simulink model "Copy_3_continuos_plant"  (R2016b)
settings: Solver=ode15s  StartTime=0.0  StopTime=300  RelTol=0.01  AbsTol=0.01
undefined symbols (not defined in the file or in its folder): deg, rad, s
libraries: simulink x12, aerolibconvert2 x4, aerolib6dof2 x2, dspsrcs4 x2, dspinverses x1
(part 1 of 2)
settings Model: Creator=Utente  LastModifiedBy=liana
settings SolverCC: MaxOrder=3  MaxConsecutiveMinStep=5  SolverJacobianMethodControl=FullAnalytical  ZeroCrossControl=DisableAll
settings DataIOCC: SaveState=on
settings OptimizationCC: BlockReduction=off  DefaultParameterBehavior=Inlined  BufferReuse=off

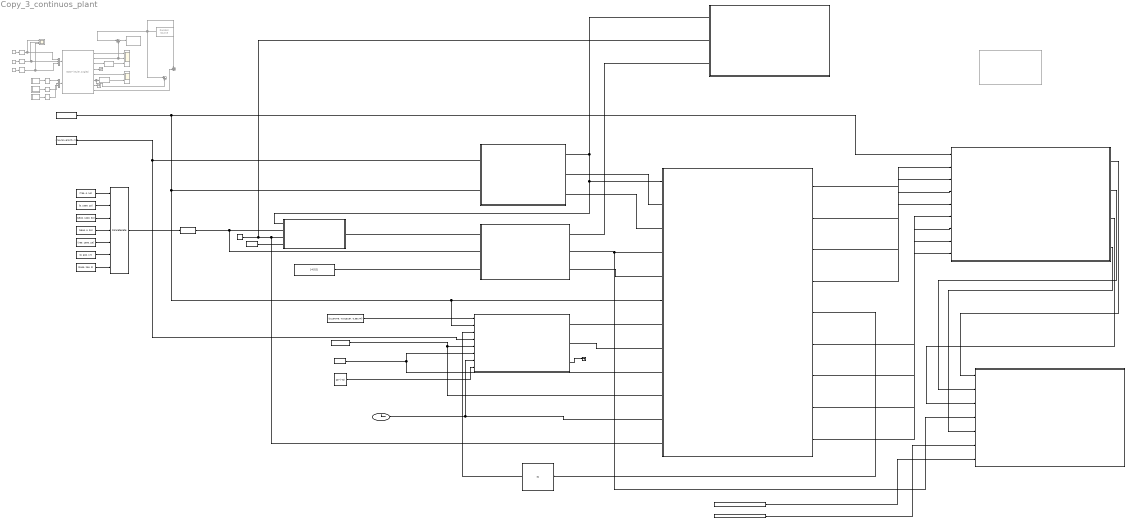
== system Copy_3_continuos_plant ==
  note: Six Degree of Freedom Motion Platform
  note: Copyright 1990-2016 The MathWorks, Inc.
  6DOF (Euler Angles) : aerolib6dof2/6DOF (Euler Angles)  Commented=on  units=Metric (MKS)  mtype=Fixed  rep=Euler Angles  xme_0=[0 0 0]  Vm_0=[0 0 0]  eul_0=[0 0 0]  pm_0=[0 0 0]  mass_0=1.0  mass_e=0.5  mass_f=2.0  inertia=eye(3)  inertia_e=eye(3)  inertia_f=2*eye(3)  k_quat=1.0  vre_flag=on
  Angle Conversion : aerolibconvert2/Angle Conversion  Commented=on  IU=rad  OU=deg
  Angular Velocity Conversion : aerolibconvert2/Angular Velocity Conversion  Commented=on  IU=rad/s  OU=deg/s
  Attitude Observer : Subsystem
  Body : Scope  Commented=on  NumInputPorts=2
  Clock : Clock
      settings: Decimation=50
  Const : Constant  Commented=on
  Const1 : Constant  Commented=on  Value=0
  Const2 : Constant  Commented=on  Value=0
  From File : FromFile  FileName=angular_velocity.mat  SampleTime=0
  From File1 : FromFile  FileName=acceleration.mat  SampleTime=0
  Fx Slider : simulink/Math Operations/Slider Gain  Commented=on  low=-1  gain=0.29496  high=1
  Fy Slider : simulink/Math Operations/Slider Gain  Commented=on  low=-1  gain=0.20144  high=1
  Fz Slider : simulink/Math Operations/Slider Gain  Commented=on  low=-1  gain=0.05036  high=1
  IC : InitialCondition  Value=[0;0;0]
  IMU data generation : Subsystem  Commented=on
  Inertial : Scope  Commented=on  NumInputPorts=3
  Kalman - Bucy Filter : Subsystem
  Kp : Constant  Value=[10 0 0; 0 10 0; 0 0 10] * 100
  Local linearization1 : Subsystem
  Math Function : Math  Operator=transpose  SaturateOnIntegerOverflow=on
  Matrix Concatenate (transponders positions) : Concatenate  NumInputs=7  Mode=Multidimensional array  ConcatenateDimension=2
  Mechanisation subsystem : Subsystem
  Mux : Mux  Commented=on  Inputs=3
  Mux1 : Mux  Commented=on  Inputs=3
  Mxx Slider : simulink/Math Operations/Slider Gain  Commented=on  low=0  gain=0  high=1
  Myy Slider : simulink/Math Operations/Slider Gain  Commented=on  low=-1  gain=0  high=1
  Mzz Slider : simulink/Math Operations/Slider Gain  Commented=on  low=-1  gain=-1  high=3
  Nonlinear algebraic transform and solution : Subsystem
  Pitch moment : Subsystem  Commented=on  mask(timed input){t=[0 3 3 4 4 5 5  7.5 7.5 8.5 8.5 9.5 9.5 10], u=[0 0  1 1 -1 -1.005 0 0 -1 -1 1 1 0 0]*3.138/2}
      mask prompts: t "time values:"; u "input values"
      mask Display: plot(t,u)
  Q matrix : Constant  Value=diag([0, 0, 0, 10^-5, 10^-3, 10^-3, 10^-3, 10^-8, 10^-8, 10^-8])
  R matrix : Constant  Value=0.25*diag([1 1 1 1 1 1])
  Random Source : dspsrcs4/Random Source  Commented=on  SrcType=Gaussian  NormMethod=Ziggurat  CltLength=12  MinVal=0  MaxVal=1  MeanVal=[0; 0; 0]  VarVal=[0.5; 0.5; 0.5]  RepMode=Not repeatable  rawSeed=1  IsInherit=off  SampMode=Continuous  SampTime=-1  SampFrame=1  DataType=Double  OutComplex=Real  OutputFrames=off
  Roll moment : Subsystem  Commented=on  mask(timed input){t=[0 1 1 2 2  10], u=[1 1 -1 -.998  0 0]*3.144/2}
      mask prompts: t "time values:"; u "input values"
      mask Display: plot(t,u)
  Scope : Scope  Commented=on  NumInputPorts=3
  Sum1 : Sum  Commented=on  Inputs=|++
  Sum2 : Sum  Commented=on  Inputs=++|
  Sum3 : Sum  Commented=on  Inputs=|++
  Terminator : Terminator
  Terminator1 : Terminator  Commented=on
  Terminator3 : Terminator  Commented=on
  Translational Motion Observer : Subsystem
  Yaw moment : Subsystem  Commented=on  mask(timed input){t=[0 6 6 7 7 8 8 10], u=[0 0  -1 -1 1 1 0 0]*3.1/2}
      mask prompts: t "time values:"; u "input values"
      mask Display: plot(t,u)
  algebraic transform - error dynamics : Subsystem
  beta : Constant  Value=100
  epsilon : Constant  Value=[1 1 1 1 1 1 1]*0.1
  ki : Constant  Value=10^(-5)
  magneto_values (Pisa) : Constant  Value=[0.237976, -0.013187, 0.39174]'
  p_n_1 : Constant  Value=[750, 0, 10]
  p_n_2 : Constant  Value=[0, 1000, 15]
  p_n_3 : Constant  Value=[1500, 1000, 30]
  p_n_4 : Constant  Value=[1500, 0, 20]
  p_n_5 : Constant  Value=[750, 1000, 25]
  p_n_6 : Constant  Value=[0, 600, 17]
  p_n_7 : Constant  Value=[2000, 200, 2]
  pos_nav file : ToFile  Commented=on  Filename=position_nav.mat  MatrixName=pos_nav  SaveFormat=Timeseries
  position_0_fixed_reference : Constant  Value=[4 5 5]
  pseudorange_measurement_model : MATLAB Function  TreatAsAtomicUnit=on
  sigma : Constant  Value=0.1
  wires:
  Clock/1 -> Translational Motion Observer/11(t), Attitude Observer/7(t)
  Nonlinear algebraic transform and solution/2(delta) -> Kalman - Bucy Filter/4(sensors measurements), Translational Motion Observer/4(delta)
  Attitude Observer/1(J) -> Translational Motion Observer/7(J)
  Attitude Observer/2(R_nb_stim) -> Translational Motion Observer/8(R_nb_stim)
  Attitude Observer/3(b_stim) -> Terminator/1
  Kp/1 -> Translational Motion Observer/10(Kp), Attitude Observer/5(Kp)
  sigma/1 -> Translational Motion Observer/9(sigma), Attitude Observer/6(sigma)
  Nonlinear algebraic transform and solution/3(C_dx) -> Translational Motion Observer/5(C_dx)
  Local linearization1/1(AL) -> Kalman - Bucy Filter/1(AL)
  Local linearization1/2(BL) -> Kalman - Bucy Filter/2(BL)
  Local linearization1/3(CL) -> Kalman - Bucy Filter/3(CL)
  pseudorange_measurement_model/1(y) -> Nonlinear algebraic transform and solution/1(y)
  Local linearization1/4(U) -> Kalman - Bucy Filter/5(U)
  epsilon/1 -> pseudorange_measurement_model/4(epsilon)
  Matrix Concatenate (transponders positions)/1 -> Math Function/1
  R matrix/1 -> Kalman - Bucy Filter/6(R)
  Q matrix/1 -> Kalman - Bucy Filter/7(Q)
  Translational Motion Observer/1(K) -> Local linearization1/2(K)
  Translational Motion Observer/2("C ") -> Local linearization1/3(C)
  Translational Motion Observer/3(" A") -> Local linearization1/4(A)
  Translational Motion Observer/4(B) -> Local linearization1/5(B)
  ki/1 -> Attitude Observer/8(Ki)
  p_n_5/1 -> Matrix Concatenate (transponders positions)/5
  p_n_4/1 -> Matrix Concatenate (transponders positions)/4
  p_n_3/1 -> Matrix Concatenate (transponders positions)/3
  p_n_2/1 -> Matrix Concatenate (transponders positions)/2
  p_n_1/1 -> Matrix Concatenate (transponders positions)/1
  Math Function/1 -> Nonlinear algebraic transform and solution/2(p), pseudorange_measurement_model/2(p_n_i)
  position_0_fixed_reference/1 -> Nonlinear algebraic transform and solution/3(p0)
  magneto_values (Pisa)/1 -> Attitude Observer/1(m_b_mag)
  p_n_6/1 -> Matrix Concatenate (transponders positions)/6
  Yaw moment/1(Out1) -> Mzz Slider/1
  Pitch moment/1(Out1) -> Myy Slider/1
  Roll moment/1(Out1) -> Mxx Slider/1
  Const2/1 -> Fz Slider/1
  Const1/1 -> Fy Slider/1
  Const/1 -> Fx Slider/1
  Mux1/1 -> 6DOF (Euler Angles)/2
  Mzz Slider/1 -> Mux1/3
  Myy Slider/1 -> Mux1/2
  Mxx Slider/1 -> Mux1/1
  Mux/1 -> 6DOF (Euler Angles)/1
  Fy Slider/1 -> Scope/2, Mux/2
  Fz Slider/1 -> Scope/3, Mux/3
  Fx Slider/1 -> Scope/1, Mux/1
  6DOF (Euler Angles)/4 -> Terminator3/1
  6DOF (Euler Angles)/7 -> Terminator1/1
  6DOF (Euler Angles)/3 -> Angle Conversion/1
  6DOF (Euler Angles)/5 -> Body/1  "Velocity in Body Axes"
  6DOF (Euler Angles)/1 -> Inertial/1  "Velocity in Inertial Axes"
  6DOF (Euler Angles)/2 -> Inertial/2, Sum1/2  "Position in Inertial Axes"
  Angle Conversion/1 -> Inertial/3  "Euler Angles"
  6DOF (Euler Angles)/6 -> Sum3/2, Angular Velocity Conversion/1
  Angular Velocity Conversion/1 -> Body/2  "Body Rotational Rates"
  6DOF (Euler Angles)/8 -> Sum2/2
  Random Source/1 -> Sum3/1, Sum2/1, Sum1/1
  Sum1/1 -> pos_nav file/1
  From File/1 -> Attitude Observer/4(w_ib), Mechanisation subsystem/1(w_ib)
  From File1/1 -> Translational Motion Observer/6(f_b_imu), Attitude Observer/2(f_b), Mechanisation subsystem/2(f_b_imu), Local linearization1/1(f_b_imu)
  p_n_7/1 -> Matrix Concatenate (transponders positions)/7
  beta/1 -> algebraic transform - error dynamics/2(beta), Translational Motion Observer/12(beta_true), pseudorange_measurement_model/3(beta)
  Mechanisation subsystem/2(v_n) -> Translational Motion Observer/2(v_n_true)
  Mechanisation subsystem/3(f_n) -> Translational Motion Observer/3(f_n_true)
  Translational Motion Observer/5(f_n_stim) -> IC/1
  Mechanisation subsystem/1(p_n) -> Translational Motion Observer/1(p_n_delta_true), pseudorange_measurement_model/1(p_n), algebraic transform - error dynamics/1(p_n_true)
  Translational Motion Observer/6(p_n_delta_err) -> Local linearization1/6(p_n_err)
  Translational Motion Observer/7(beta_err) -> Local linearization1/7(beta_err)
  Translational Motion Observer/8(v_n_err) -> Local linearization1/8(v_n_err)
  Translational Motion Observer/9(f_n_err) -> Local linearization1/9(f_n_err)
  Nonlinear algebraic transform and solution/1(x_at) -> algebraic transform - error dynamics/3(x_at)
  IC/1 -> Attitude Observer/3(f_n_stim)

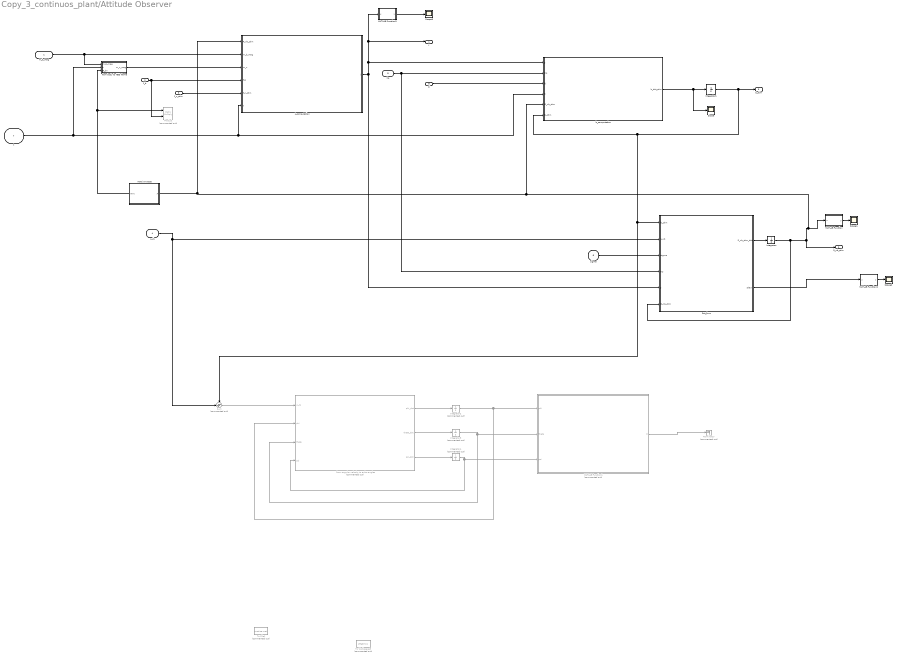
== system Copy_3_continuos_plant/Attitude Observer ==
  m_b_mag : Inport
  f_b : Inport  Port=2
  f_n_stim : Inport  Port=3
  w_ib : Inport  Port=4
  Kp : Inport  Port=5
  sigma : Inport  Port=6
  t : Inport  Port=7
  Ki : Inport  Port=8
  Integrator : Integrator  InitialCondition=eye(3)  AbsoluteTolerance=0.000000000001
  Integrator1 : Integrator  InitialCondition=0.02  UpperSaturationLimit=100  LowerSaturationLimit=-100  AbsoluteTolerance=0.0000001
  Integrator2 : Integrator  Commented=on
  Integrator3 : Integrator  Commented=on
  Integrator4 : Integrator  Commented=on
  J_computation : Subsystem
  MATLAB Function : MATLAB Function  TreatAsAtomicUnit=on
  MATLAB Function1 : MATLAB Function  Commented=on  TreatAsAtomicUnit=on
  MATLAB Function2 : MATLAB Function  TreatAsAtomicUnit=on
  MATLAB Function3 : MATLAB Function  TreatAsAtomicUnit=on
  Product : Product  Commented=on  Multiplication=Matrix(*)
  Rot_func : MATLAB Function  TreatAsAtomicUnit=on
  Scope{,1..3} (4 alike) : Scope
  Sum : Sum  Commented=on  Inputs=-+|
  Terminator : Terminator  Commented=on
  To File1 : ToFile  Commented=on  Filename=matrice.mat  MatrixName=m  SaveFormat=Timeseries
  To Workspace5 : ToWorkspace  Commented=on  VariableName=JMatrix1  SaveFormat=Timeseries  SampleTime=-1
  b_computation : MATLAB Function  TreatAsAtomicUnit=on
  from angular velocity to euler angles : MATLAB Function  Commented=on  TreatAsAtomicUnit=on
  from body to NED frame : MATLAB Function  TreatAsAtomicUnit=on
  matrixInverse : MATLAB Function  TreatAsAtomicUnit=on
  J : Outport
  R_nb_stim : Outport  Port=2
  b_stim : Outport  Port=3
  wires:
  m_b_mag/1 -> from body to NED frame/1(m_b_mag), J_computation/2(m_b_mag)
  from body to NED frame/1(m_n_mag) -> J_computation/3(m_n)
  f_b/1 -> Product/2, J_computation/4(f_b)
  J_computation/1(J) -> MATLAB Function3/1(u), J/1, b_computation/1(J), Rot_func/5(J)
  Kp/1 -> Rot_func/4(Kp), b_computation/2(Kp)
  Ki/1 -> b_computation/3(ki)
  sigma/1 -> Rot_func/3(sigma)
  w_ib/1 -> Sum/2, Rot_func/2(w_ib)
  t/1 -> from body to NED frame/2(t), b_computation/4(t), J_computation/6(t)
  b_computation/1(b_dot_stim) -> Scope/1, Integrator1/1
  matrixInverse/1(AInv) -> from body to NED frame/3(R_bn), Product/1
  MATLAB Function/1(y) -> Scope1/1
  Sum/1 -> from angular velocity to euler angles/1(w_ib)
  from angular velocity to euler angles/1(phi_dot) -> Integrator2/1
  from angular velocity to euler angles/2(theta_dot) -> Integrator3/1
  from angular velocity to euler angles/3(psi_dot) -> Integrator4/1
  Integrator3/1 -> MATLAB Function1/2(theta), from angular velocity to euler angles/3(theta)
  Integrator4/1 -> MATLAB Function1/3(psi), from angular velocity to euler angles/4(psi)
  Integrator2/1 -> from angular velocity to euler angles/2(phi), MATLAB Function1/1(phi)
  MATLAB Function2/1(y) -> Scope2/1
  Rot_func/2(Skew) -> MATLAB Function2/1(u)
  Integrator1/1 -> b_computation/6(b_stim), Sum/1, Rot_func/1(b_stim), b_stim/1
  MATLAB Function1/1(R) -> Terminator/1
  MATLAB Function3/1(y) -> Scope3/1
  Rot_func/1(R_nb_stim_dot) -> Integrator/1
  Integrator/1 -> Rot_func/6(R_nb_stim), J_computation/1(R_nb_stim), matrixInverse/1(A), b_computation/5(R_nb_stim), MATLAB Function/1(u), R_nb_stim/1
  f_n_stim/1 -> J_computation/5(f_n_stim)

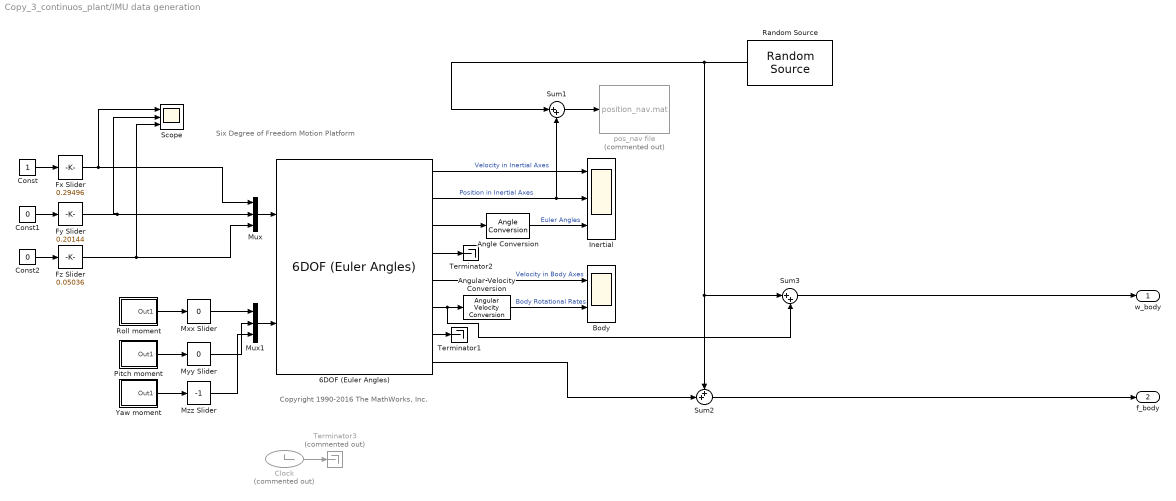
== system Copy_3_continuos_plant/IMU data generation ==
  note: Six Degree of Freedom Motion Platform
  note: Copyright 1990-2016 The MathWorks, Inc.
  6DOF (Euler Angles) : aerolib6dof2/6DOF (Euler Angles)  units=Metric (MKS)  mtype=Fixed  rep=Euler Angles  xme_0=[0 0 0]  Vm_0=[0 0 0]  eul_0=[0 0 0]  pm_0=[0 0 0]  mass_0=1.0  mass_e=0.5  mass_f=2.0  inertia=eye(3)  inertia_e=eye(3)  inertia_f=2*eye(3)  k_quat=1.0  vre_flag=on
  Angle Conversion : aerolibconvert2/Angle Conversion  IU=rad  OU=deg
  Angular Velocity Conversion : aerolibconvert2/Angular Velocity Conversion  IU=rad/s  OU=deg/s
  Body : Scope  NumInputPorts=2
  Clock : Clock  Commented=on
      settings: Decimation=100
  Const : Constant
  Const1 : Constant  Value=0
  Const2 : Constant  Value=0
  Fx Slider : simulink/Math Operations/Slider Gain  low=-1  gain=0.29496  high=1
  Fy Slider : simulink/Math Operations/Slider Gain  low=-1  gain=0.20144  high=1
  Fz Slider : simulink/Math Operations/Slider Gain  low=-1  gain=0.05036  high=1
  Inertial : Scope  NumInputPorts=3
  Mux : Mux  Inputs=3
  Mux1 : Mux  Inputs=3
  Mxx Slider : simulink/Math Operations/Slider Gain  low=0  gain=0  high=1
  Myy Slider : simulink/Math Operations/Slider Gain  low=-1  gain=0  high=1
  Mzz Slider : simulink/Math Operations/Slider Gain  low=-1  gain=-1  high=3
  Pitch moment : Subsystem  mask(timed input){t=[0 3 3 4 4 5 5  7.5 7.5 8.5 8.5 9.5 9.5 10], u=[0 0  1 1 -1 -1.005 0 0 -1 -1 1 1 0 0]*3.138/2}
      mask prompts: t "time values:"; u "input values"
      mask Display: plot(t,u)
  Random Source : dspsrcs4/Random Source  SrcType=Gaussian  NormMethod=Ziggurat  CltLength=12  MinVal=0  MaxVal=1  MeanVal=[0; 0; 0]  VarVal=[0.5; 0.5; 0.5]  RepMode=Not repeatable  rawSeed=1  IsInherit=off  SampMode=Continuous  SampTime=-1  SampFrame=1  DataType=Double  OutComplex=Real  OutputFrames=off
  Roll moment : Subsystem  mask(timed input){t=[0 1 1 2 2  10], u=[1 1 -1 -.998  0 0]*3.144/2}
      mask prompts: t "time values:"; u "input values"
      mask Display: plot(t,u)
  Scope : Scope  NumInputPorts=3
  Sum1 : Sum  Inputs=|++
  Sum2 : Sum  Inputs=++|
  Sum3 : Sum  Inputs=|++
  Terminator1 : Terminator
  Terminator2 : Terminator
  Terminator3 : Terminator  Commented=on
  Yaw moment : Subsystem  mask(timed input){t=[0 6 6 7 7 8 8 10], u=[0 0  -1 -1 1 1 0 0]*3.1/2}
      mask prompts: t "time values:"; u "input values"
      mask Display: plot(t,u)
  pos_nav file : ToFile  Commented=on  Filename=position_nav.mat  MatrixName=pos_nav  SaveFormat=Timeseries
  w_body : Outport
  f_body : Outport  Port=2
  wires:
  Yaw moment/1(Out1) -> Mzz Slider/1
  Pitch moment/1(Out1) -> Myy Slider/1
  Roll moment/1(Out1) -> Mxx Slider/1
  Const2/1 -> Fz Slider/1
  Const1/1 -> Fy Slider/1
  Const/1 -> Fx Slider/1
  Clock/1 -> Terminator3/1
  Mux1/1 -> 6DOF (Euler Angles)/2
  Mzz Slider/1 -> Mux1/3
  Myy Slider/1 -> Mux1/2
  Mxx Slider/1 -> Mux1/1
  Mux/1 -> 6DOF (Euler Angles)/1
  Fy Slider/1 -> Scope/2, Mux/2
  Fz Slider/1 -> Scope/3, Mux/3
  Fx Slider/1 -> Scope/1, Mux/1
  6DOF (Euler Angles)/4 -> Terminator2/1
  6DOF (Euler Angles)/7 -> Terminator1/1
  6DOF (Euler Angles)/3 -> Angle Conversion/1
  6DOF (Euler Angles)/5 -> Body/1  "Velocity in Body Axes"
  6DOF (Euler Angles)/1 -> Inertial/1  "Velocity in Inertial Axes"
  6DOF (Euler Angles)/2 -> Inertial/2, Sum1/2  "Position in Inertial Axes"
  Angle Conversion/1 -> Inertial/3  "Euler Angles"
  6DOF (Euler Angles)/6 -> Sum3/2, Angular Velocity Conversion/1
  Angular Velocity Conversion/1 -> Body/2  "Body Rotational Rates"
  6DOF (Euler Angles)/8 -> Sum2/2
  Random Source/1 -> Sum1/1, Sum2/1, Sum3/1
  Sum1/1 -> pos_nav file/1
  Sum2/1 -> f_body/1
  Sum3/1 -> w_body/1

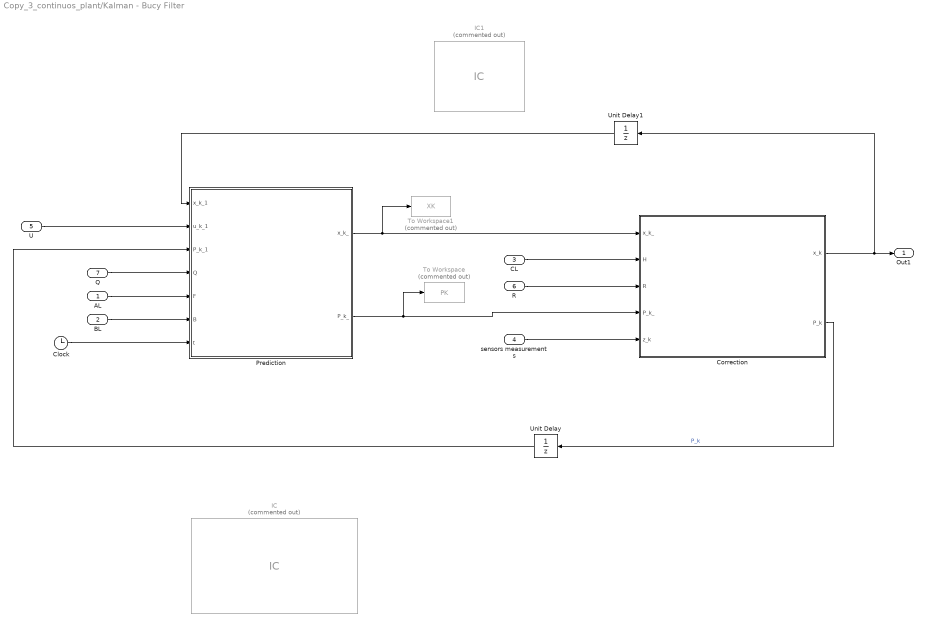
== system Copy_3_continuos_plant/Kalman - Bucy Filter ==
  AL : Inport
  BL : Inport  Port=2
  CL : Inport  Port=3
  sensors measurements : Inport  Port=4
  U : Inport  Port=5
  R : Inport  Port=6
  Q : Inport  Port=7
  Clock : Clock
  Correction : MATLAB Function  TreatAsAtomicUnit=on
  IC : InitialCondition  Commented=on  Value=diag([3*(10^3),3*(10^3),3*(10^3),3*(10^3),10,10,10,0.01,0.01,0.01])
  IC1 : InitialCondition  Commented=on  Value=[0;0;0;0;0;0;0;0;0;0]
  Prediction : MATLAB Function  TreatAsAtomicUnit=on
  To Workspace : ToWorkspace  Commented=on  VariableName=PK  SaveFormat=Timeseries  SampleTime=-1
  To Workspace1 : ToWorkspace  Commented=on  VariableName=XK  SaveFormat=Timeseries  SampleTime=-1
  Unit Delay : UnitDelay  SampleTime=-1
  Unit Delay1 : UnitDelay  SampleTime=-1
  Out1 : Outport
  wires:
  Prediction/2(P_k_) -> To Workspace/1, Correction/4(P_k_)
  Prediction/1(x_k_) -> To Workspace1/1, Correction/1(x_k_)
  Correction/1(x_k) -> Unit Delay1/1, Out1/1
  AL/1 -> Prediction/5(F)
  CL/1 -> Correction/2(H)
  Clock/1 -> Prediction/7(t)
  Q/1 -> Prediction/4(Q)
  sensors measurements/1 -> Correction/5(z_k)
  BL/1 -> Prediction/6(B)
  U/1 -> Prediction/2(u_k_1)
  R/1 -> Correction/3(R)
  Unit Delay/1 -> Prediction/3(P_k_1)
  Correction/2(P_k) -> Unit Delay/1  "P_k"
  Unit Delay1/1 -> Prediction/1(x_k_1)

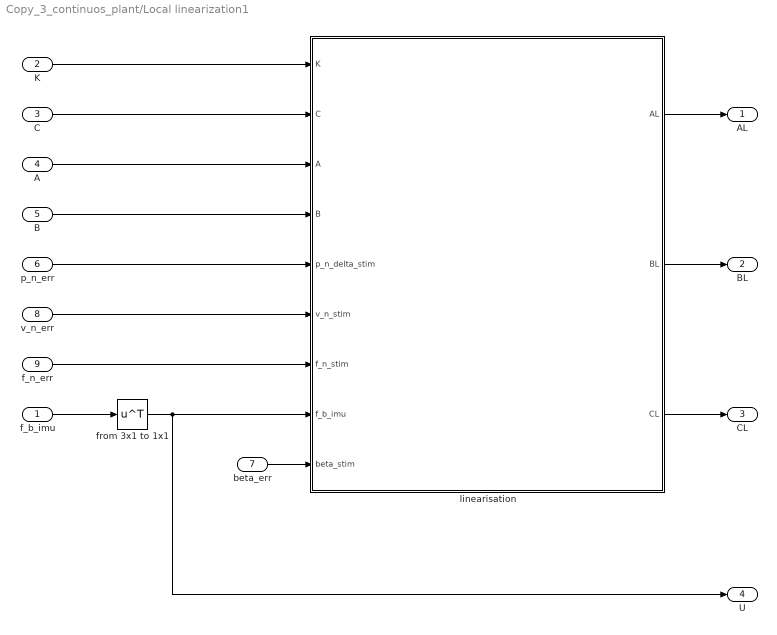
== system Copy_3_continuos_plant/Local linearization1 ==
  f_b_imu : Inport
  K : Inport  Port=2
  C : Inport  Port=3
  A : Inport  Port=4
  B : Inport  Port=5
  p_n_err : Inport  Port=6
  beta_err : Inport  Port=7
  v_n_err : Inport  Port=8
  f_n_err : Inport  Port=9
  from 3x1 to 1x1 : Math  Operator=transpose  SaturateOnIntegerOverflow=on
  linearisation : MATLAB Function  TreatAsAtomicUnit=on
  AL : Outport
  BL : Outport  Port=2
  CL : Outport  Port=3
  U : Outport  Port=4
  wires:
  linearisation/1(AL) -> AL/1
  linearisation/2(BL) -> BL/1
  linearisation/3(CL) -> CL/1
  K/1 -> linearisation/1(K)
  C/1 -> linearisation/2(C)
  A/1 -> linearisation/3(A)
  B/1 -> linearisation/4(B)
  p_n_err/1 -> linearisation/5(p_n_delta_stim)
  beta_err/1 -> linearisation/9(beta_stim)
  v_n_err/1 -> linearisation/6(v_n_stim)
  f_b_imu/1 -> from 3x1 to 1x1/1
  f_n_err/1 -> linearisation/7(f_n_stim)
  from 3x1 to 1x1/1 -> U/1, linearisation/8(f_b_imu)

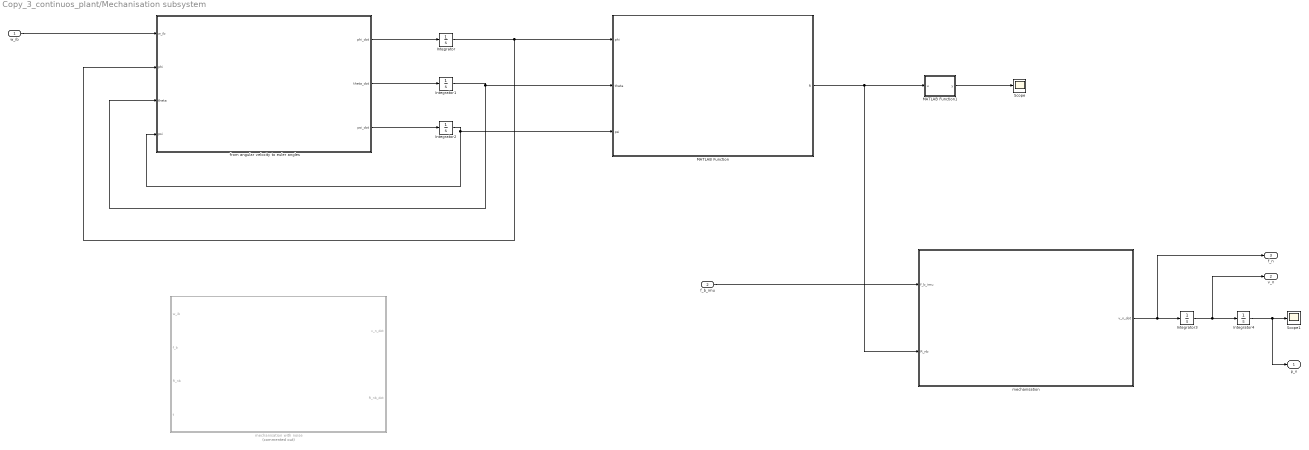
== system Copy_3_continuos_plant/Mechanisation subsystem ==
  w_ib : Inport
  f_b_imu : Inport  Port=2
  Integrator : Integrator  AbsoluteTolerance=0.001
  Integrator1 : Integrator
  Integrator2 : Integrator  AbsoluteTolerance=0.001
  Integrator3 : Integrator
  Integrator4 : Integrator
  MATLAB Function : MATLAB Function  TreatAsAtomicUnit=on
  MATLAB Function1 : MATLAB Function  TreatAsAtomicUnit=on
  Scope : Scope
  Scope1 : Scope
  from angular velocity to euler angles : MATLAB Function  TreatAsAtomicUnit=on
  mechanisation : MATLAB Function  TreatAsAtomicUnit=on
  mechanisation with noise : MATLAB Function  Commented=on  TreatAsAtomicUnit=on
  p_n : Outport
  v_n : Outport  Port=2
  f_n : Outport  Port=3
  wires:
  w_ib/1 -> from angular velocity to euler angles/1(w_ib)
  from angular velocity to euler angles/1(phi_dot) -> Integrator/1
  from angular velocity to euler angles/2(theta_dot) -> Integrator1/1
  from angular velocity to euler angles/3(psi_dot) -> Integrator2/1
  Integrator1/1 -> MATLAB Function/2(theta), from angular velocity to euler angles/3(theta)
  Integrator2/1 -> MATLAB Function/3(psi), from angular velocity to euler angles/4(psi)
  Integrator/1 -> from angular velocity to euler angles/2(phi), MATLAB Function/1(phi)
  MATLAB Function/1(R) -> mechanisation/2(R_nb), MATLAB Function1/1(u)
  MATLAB Function1/1(y) -> Scope/1
  f_b_imu/1 -> mechanisation/1(f_b_imu)
  Integrator3/1 -> v_n/1, Integrator4/1
  Integrator4/1 -> p_n/1, Scope1/1
  mechanisation/1(v_n_dot) -> f_n/1, Integrator3/1

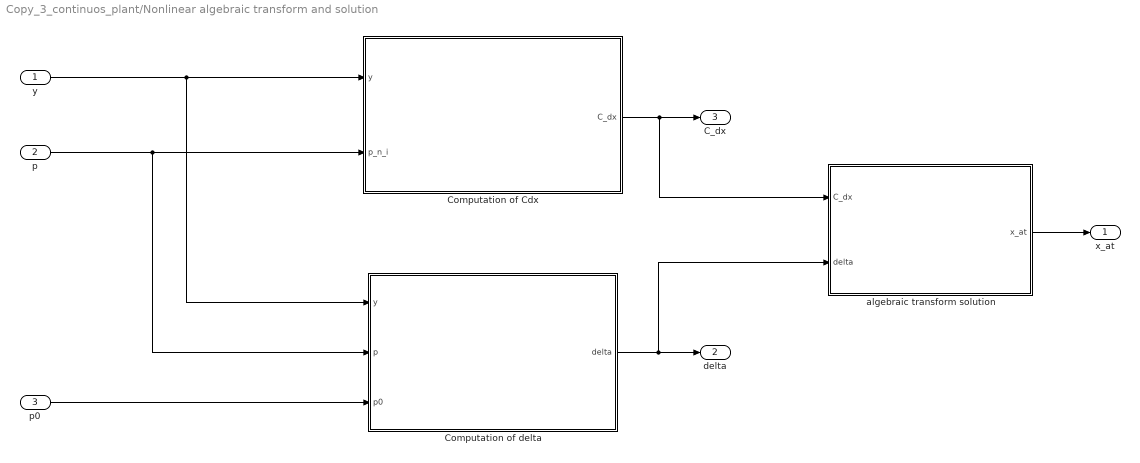
== system Copy_3_continuos_plant/Nonlinear algebraic transform and solution ==
  y : Inport
  p : Inport  Port=2
  p0 : Inport  Port=3
  Computation of Cdx : MATLAB Function  TreatAsAtomicUnit=on
  Computation of delta : MATLAB Function  TreatAsAtomicUnit=on
  algebraic transform solution : MATLAB Function  TreatAsAtomicUnit=on
  x_at : Outport
  delta : Outport  Port=2
  C_dx : Outport  Port=3
  wires:
  y/1 -> Computation of delta/1(y), Computation of Cdx/1(y)
  p/1 -> Computation of delta/2(p), Computation of Cdx/2(p_n_i)
  p0/1 -> Computation of delta/3(p0)
  Computation of delta/1(delta) -> algebraic transform solution/2(delta), delta/1
  Computation of Cdx/1(C_dx) -> algebraic transform solution/1(C_dx), C_dx/1
  algebraic transform solution/1(x_at) -> x_at/1

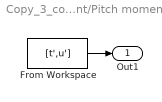
== system Copy_3_continuos_plant/Pitch moment ==
  From Workspace : FromWorkspace  VariableName=[t',u']  SampleTime=0
  Out1 : Outport
  wires:
  From Workspace/1 -> Out1/1

== system Copy_3_continuos_plant/Roll moment ==
  From Workspace : FromWorkspace  VariableName=[t',u']  SampleTime=0
  Out1 : Outport
  wires:
  From Workspace/1 -> Out1/1

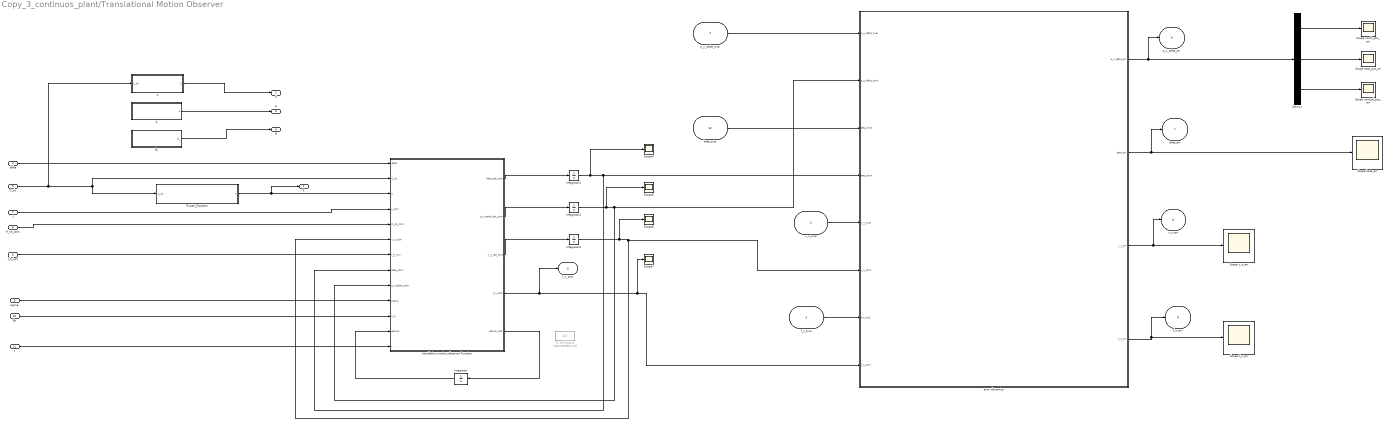
== system Copy_3_continuos_plant/Translational Motion Observer ==
  p_n_delta_true : Inport
  v_n_true : Inport  Port=2
  f_n_true : Inport  Port=3
  delta : Inport  Port=4
  C_dx : Inport  Port=5
  f_b_imu : Inport  Port=6
  J : Inport  Port=7
  R_nb_stim : Inport  Port=8
  sigma : Inport  Port=9
  Kp : Inport  Port=10
  t : Inport  Port=11
  beta_true : Inport  Port=12
  A : MATLAB Function  TreatAsAtomicUnit=on
  B_ : MATLAB Function  TreatAsAtomicUnit=on
  C : MATLAB Function  TreatAsAtomicUnit=on
  Demux : Demux  Outputs=3
  Integrator : Integrator  AbsoluteTolerance=0.01
  Integrator1 : Integrator  InitialCondition=100  AbsoluteTolerance=0.00001
  Integrator2 : Integrator  AbsoluteTolerance=0.01
  Integrator3 : Integrator  AbsoluteTolerance=0.01
  Riccati_Equation : Subsystem
  Scope beta_err : Scope
  Scope f_n_err : Scope
  Scope v_n_err : Scope
  Scope east_pos_err : Scope
  Scope north_pos_err : Scope
  Scope vertical_pos_err : Scope
  Scope{4..7} (4 alike) : Scope
  To Workspace : ToWorkspace  Commented=on  VariableName=KO  SaveFormat=Timeseries  SampleTime=-1
  error dynamics : MATLAB Function  TreatAsAtomicUnit=on
  translation_motion_observer Function : MATLAB Function  TreatAsAtomicUnit=on
  K : Outport
  "C " : Outport  Port=2
  " A" : Outport  Port=3
  B : Outport  Port=4
  f_n_stim : Outport  Port=5
  p_n_delta_err : Outport  Port=6
  beta_err : Outport  Port=7
  v_n_err : Outport  Port=8
  f_n_err : Outport  Port=9
  wires:
  translation_motion_observer Function/4(f_n_stim) -> f_n_stim/1, Scope7/1, error dynamics/8(f_n_stim)
  translation_motion_observer Function/3(v_n_dot_stim) -> Integrator3/1
  translation_motion_observer Function/2(p_n_delta_dot_stim) -> Integrator2/1
  C_dx/1 -> C/1(C_dx), Riccati_Equation/1(C_dx), translation_motion_observer Function/2(C_dx)
  J/1 -> translation_motion_observer Function/4(J_stim)
  R_nb_stim/1 -> translation_motion_observer Function/5(R_nb_stim)
  delta/1 -> translation_motion_observer Function/1(delta)
  f_b_imu/1 -> translation_motion_observer Function/7(f_b_imu)
  sigma/1 -> translation_motion_observer Function/10(sigma)
  Kp/1 -> translation_motion_observer Function/11(K_p)
  A/1(A) -> " A"/1
  C/1(C) -> "C "/1
  Riccati_Equation/1(K) -> K/1, translation_motion_observer Function/3(K)
  B_/1(B_) -> B/1
  t/1 -> translation_motion_observer Function/13(t)
  Integrator3/1 -> Scope6/1, error dynamics/6(v_n_stim), translation_motion_observer Function/6(v_n_stim)
  translation_motion_observer Function/1(beta_dot_stim) -> Integrator1/1
  Integrator/1 -> translation_motion_observer Function/12(epsilon)
  Integrator1/1 -> Scope4/1, translation_motion_observer Function/8(beta_stim), error dynamics/4(beta_stim)
  translation_motion_observer Function/5(epsilon_dot) -> Integrator/1
  Integrator2/1 -> Scope5/1, error dynamics/2(p_n_delta_stim), translation_motion_observer Function/9(p_n_delta_stim)
  p_n_delta_true/1 -> error dynamics/1(p_n_delta_true)
  beta_true/1 -> error dynamics/3(beta_true)
  v_n_true/1 -> error dynamics/5(v_n_true)
  f_n_true/1 -> error dynamics/7(f_n_true)
  error dynamics/2(beta_err) -> beta_err/1, Scope beta_err/1
  error dynamics/4(f_n_err) -> f_n_err/1, Scope f_n_err/1
  error dynamics/3(v_n_err) -> v_n_err/1, Scope v_n_err/1
  error dynamics/1(p_n_delta_err) -> Demux/1, p_n_delta_err/1
  Demux/1 -> Scope north_pos_err/1
  Demux/2 -> Scope east_pos_err/1
  Demux/3 -> Scope vertical_pos_err/1

== system Copy_3_continuos_plant/Yaw moment ==
  From Workspace : FromWorkspace  VariableName=[t',u']  SampleTime=0
  Out1 : Outport
  wires:
  From Workspace/1 -> Out1/1

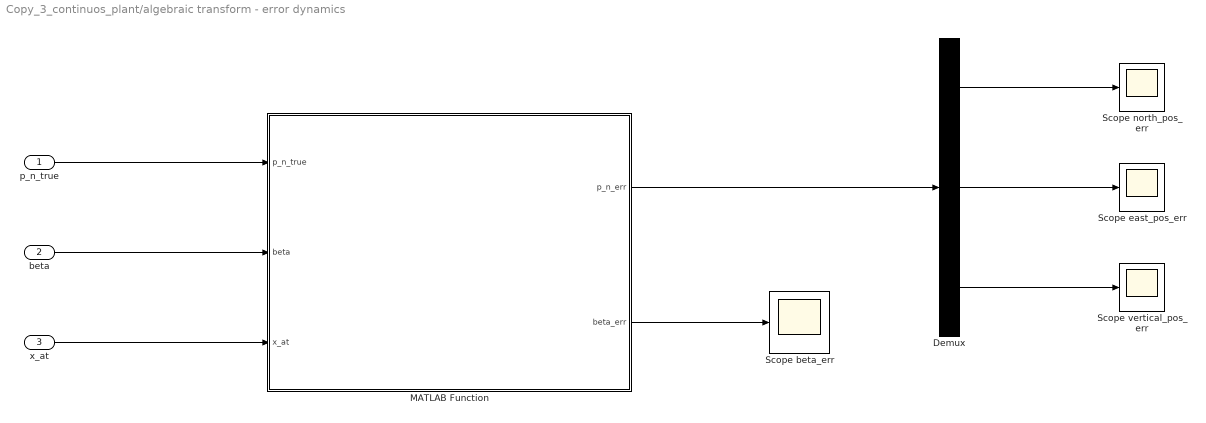
== system Copy_3_continuos_plant/algebraic transform - error dynamics ==
  p_n_true : Inport
  beta : Inport  Port=2
  x_at : Inport  Port=3
  Demux : Demux  Outputs=3
  MATLAB Function : MATLAB Function  TreatAsAtomicUnit=on
  Scope beta_err : Scope
  Scope east_pos_err : Scope
  Scope north_pos_err : Scope
  Scope vertical_pos_err : Scope
  wires:
  p_n_true/1 -> MATLAB Function/1(p_n_true)
  beta/1 -> MATLAB Function/2(beta)
  x_at/1 -> MATLAB Function/3(x_at)
  MATLAB Function/2(beta_err) -> Scope beta_err/1
  MATLAB Function/1(p_n_err) -> Demux/1
  Demux/1 -> Scope north_pos_err/1
  Demux/2 -> Scope east_pos_err/1
  Demux/3 -> Scope vertical_pos_err/1

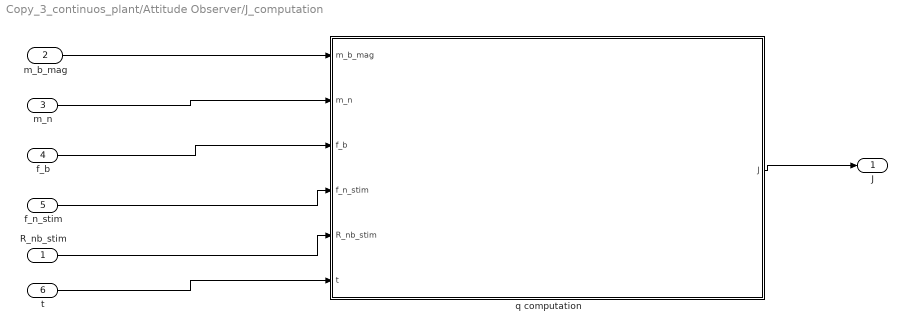
== system Copy_3_continuos_plant/Attitude Observer/J_computation ==
  R_nb_stim : Inport
  m_b_mag : Inport  Port=2
  m_n : Inport  Port=3
  f_b : Inport  Port=4
  f_n_stim : Inport  Port=5
  t : Inport  Port=6
  q computation : MATLAB Function  TreatAsAtomicUnit=on
  J : Outport
  wires:
  m_n/1 -> q computation/2(m_n)
  f_n_stim/1 -> q computation/4(f_n_stim)
  m_b_mag/1 -> q computation/1(m_b_mag)
  f_b/1 -> q computation/3(f_b)
  q computation/1(J) -> J/1
  R_nb_stim/1 -> q computation/5(R_nb_stim)
  t/1 -> q computation/6(t)

== system Copy_3_continuos_plant/IMU data generation/Pitch moment ==
  From Workspace : FromWorkspace  VariableName=[t',u']  SampleTime=0
  Out1 : Outport
  wires:
  From Workspace/1 -> Out1/1

== system Copy_3_continuos_plant/IMU data generation/Roll moment ==
  From Workspace : FromWorkspace  VariableName=[t',u']  SampleTime=0
  Out1 : Outport
  wires:
  From Workspace/1 -> Out1/1

== system Copy_3_continuos_plant/IMU data generation/Yaw moment ==
  From Workspace : FromWorkspace  VariableName=[t',u']  SampleTime=0
  Out1 : Outport
  wires:
  From Workspace/1 -> Out1/1

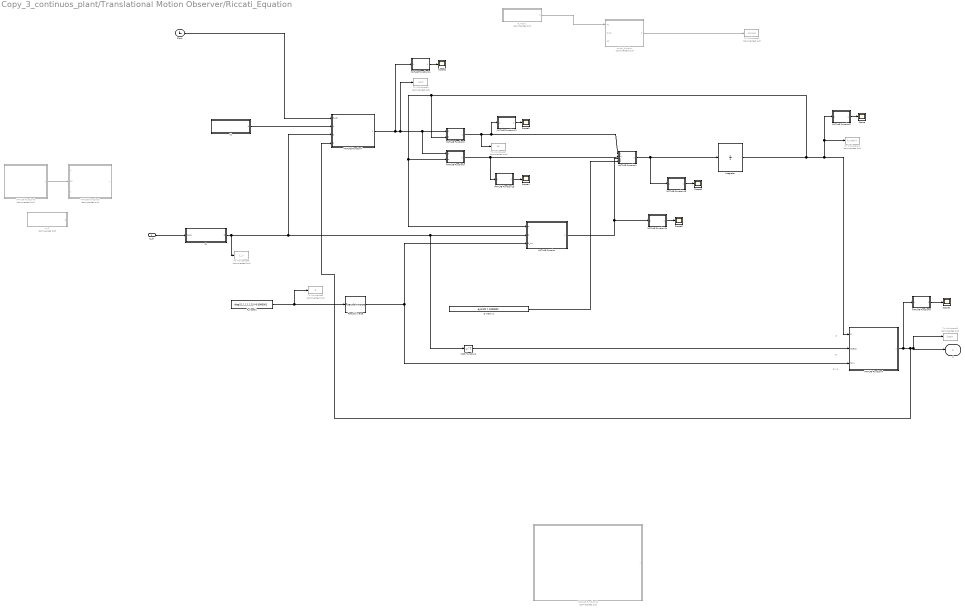
== system Copy_3_continuos_plant/Translational Motion Observer/Riccati_Equation ==
  note: R^-1
  note: C'
  note: P
  C_dx : Inport
  A1 : MATLAB Function  TreatAsAtomicUnit=on
  C_ : MATLAB Function  TreatAsAtomicUnit=on
  Clock : Clock
  Integrator : Integrator  InitialCondition=eye(10)*10  AbsoluteTolerance=0.000001
  MATLAB Function : MATLAB Function  TreatAsAtomicUnit=on
  MATLAB Function1 : MATLAB Function  TreatAsAtomicUnit=on
  MATLAB Function10 : MATLAB Function  Commented=on  TreatAsAtomicUnit=on
  MATLAB Function11 : MATLAB Function  TreatAsAtomicUnit=on
  MATLAB Function12 : MATLAB Function  TreatAsAtomicUnit=on
  MATLAB Function13 : MATLAB Function  TreatAsAtomicUnit=on
  MATLAB Function14 : MATLAB Function  TreatAsAtomicUnit=on
  MATLAB Function16 : MATLAB Function  TreatAsAtomicUnit=on
  MATLAB Function2 : MATLAB Function  TreatAsAtomicUnit=on
  MATLAB Function3 : MATLAB Function  TreatAsAtomicUnit=on
  MATLAB Function4 : MATLAB Function  TreatAsAtomicUnit=on
  MATLAB Function5 : MATLAB Function  TreatAsAtomicUnit=on
  MATLAB Function6 : MATLAB Function  TreatAsAtomicUnit=on
  MATLAB Function7 : MATLAB Function  TreatAsAtomicUnit=on
  MATLAB Function8 : MATLAB Function  Commented=on  TreatAsAtomicUnit=on
  MATLAB Function9 : MATLAB Function  Commented=on  TreatAsAtomicUnit=on
  Math Function1 : Math  Operator=transpose  SaturateOnIntegerOverflow=on
  "P_matrix " : MATLAB Function  Commented=on  TreatAsAtomicUnit=on
  Pseudoinverse : dspinverses/Pseudoinverse  wanterr=off  SimulateUsing=Interpreted execution
  Q matrix1 : Constant  Value=eye(10) * 1000000
  R_riccati1 : Constant  Value=diag([1,1,1,1,1,1])*0.0000001  VectorParams1D=off
  Scope{,1..6} (7 alike) : Scope
  To Workspace1 : ToWorkspace  Commented=on  VariableName=P_matrix  SampleTime=-1
  To Workspace2 : ToWorkspace  Commented=on  VariableName=simout  SaveFormat=Timeseries  SampleTime=-1
  To Workspace3 : ToWorkspace  Commented=on  VariableName=Kgain  SaveFormat=Timeseries  SampleTime=-1
  To Workspace5 : ToWorkspace  Commented=on  VariableName=R  SaveFormat=Timeseries  SampleTime=-1
  To Workspace7 : ToWorkspace  Commented=on  VariableName=PA  SaveFormat=Timeseries  SampleTime=-1
  To Workspace8 : ToWorkspace  Commented=on  VariableName=C_n  SaveFormat=Timeseries  SampleTime=-1
  To Workspace9 : ToWorkspace  Commented=on  VariableName=AKC  SaveFormat=Timeseries  SampleTime=-1
  myC : MATLAB Function  Commented=on  TreatAsAtomicUnit=on
  switch_function : MATLAB Function  Commented=on  TreatAsAtomicUnit=on
  K : Outport
  wires:
  R_riccati1/1 -> Pseudoinverse/1, To Workspace5/1
  Math Function1/1 -> MATLAB Function4/2(Ctrasp)
  MATLAB Function2/1(y) -> To Workspace7/1, MATLAB Function12/1(u), MATLAB Function1/1(X)
  MATLAB Function3/1(y) -> MATLAB Function13/1(u), MATLAB Function1/2(W)
  MATLAB Function/1(y) -> MATLAB Function14/1(u), MATLAB Function1/3(Z)
  MATLAB Function1/1(y) -> MATLAB Function16/1(u), Integrator/1
  C_dx/1 -> C_/1(C_dx)
  Clock/1 -> MATLAB Function7/1(clock)
  "P_matrix "/1(P) -> switch_function/1(P1)
  switch_function/1(P) -> To Workspace2/1
  Integrator/1 -> MATLAB Function4/1(P), MATLAB Function5/1(u), To Workspace1/1, MATLAB Function2/2(P), MATLAB Function3/2(P), MATLAB Function/1(P)
  MATLAB Function5/1(y) -> Scope/1
  MATLAB Function6/1(y) -> Scope1/1
  MATLAB Function8/1(y) -> MATLAB Function9/2(CK)
  MATLAB Function4/1(y) -> MATLAB Function6/1(u), MATLAB Function7/4(K), K/1, To Workspace3/1
  A1/1(A) -> MATLAB Function7/2(A)
  C_/1(C) -> To Workspace8/1, MATLAB Function7/3(C), Math Function1/1, MATLAB Function/2(C)
  MATLAB Function7/1(y) -> MATLAB Function11/1(u), To Workspace9/1, MATLAB Function3/1(A), MATLAB Function2/1(A)
  MATLAB Function11/1(y) -> Scope2/1
  MATLAB Function12/1(y) -> Scope3/1
  MATLAB Function13/1(y) -> Scope4/1
  MATLAB Function14/1(y) -> Scope5/1
  Pseudoinverse/1 -> MATLAB Function4/3(Rinv), MATLAB Function/3(R_inv)
  MATLAB Function16/1(y) -> Scope6/1
  Q matrix1/1 -> MATLAB Function1/4(Q)

== matlab function Copy_3_continuos_plant/Translational Motion Observer/Riccati_Equation/MATLAB Function ==
  data: P input; y output; C input; R_inv input
function y = fcn(P,C,R_inv)

y = - P * C' * R_inv * C * P;

end

== matlab function Copy_3_continuos_plant/Attitude Observer/J_computation/q computation ==
  data: m_b_mag input; m_n input; f_b input; f_n_stim input size=3; J output; R_nb_stim input size=[3,3]; t input
function J  = qEfunc(m_b_mag, m_n, f_b, f_n_stim, R_nb_stim, t)

% if t <= 1
%     R_nb_stim = eye(3);
% end

g_n = [0.1 0.1 9.81]';

q1_b = m_b_mag/norm(m_b_mag,2);
q2_b = f_b/norm(g_n,2);

q1_n = m_n/norm(m_n,2);
q2_n = f_n_stim/norm(g_n,2);


E_b = [q1_b, skew(q1_b)*q2_b, (skew(q1_b)*skew(q1_b))*q2_b];
E_n = [q1_n, skew(q1_n)*q2_n, (skew(q1_n)*skew(q1_n))*q2_n];

J = (E_n - R_nb_stim * E_b) * (E_b');

end

== matlab function Copy_3_continuos_plant/Kalman - Bucy Filter/Prediction ==
  data: x_k_1 input size=[10, 1]; x_k_ output; u_k_1 input; P_k_1 input size=[10,10]; Q input; F input; B input; P_k_ output; t input
function [x_k_, P_k_] = prediction(x_k_1, u_k_1, P_k_1, Q, F,B, t)

    % initial value of x_k_1
    if t == 0
        x_k_1 = zeros(10,1);
%         P_k_1 = eye(10);
    end

    x_k_ = F * x_k_1 + B * u_k_1';
    
    P_k_ = F * P_k_1 * F' + Q;
    

end

== matlab function Copy_3_continuos_plant/Translational Motion Observer/Riccati_Equation/MATLAB Function1 ==
  data: X input; y output size=[10,10]; W input; Z input; Q input
function y = fcn(X,W,Z,Q)

y =  X + W + Z + Q;
% y = Z + Q;

end

== matlab function Copy_3_continuos_plant/Mechanisation subsystem/mechanisation with noise ==
  data: w_ib input; f_b input; v_n_dot output; R_nb_dot output; R_nb input; t input
function [v_n_dot, R_nb_dot] = mechanisation(w_ib, f_b, R_nb, t)



g_n = [0.1 0.1 9.81]';

% w_ib = size(3,1);

if t == 0
    v_n_dot = zeros(3,1);
    R_nb_dot = eye(3);
    R_nb = eye(3);
end

Skew = skew(w_ib);


%p_dot = v_n;

v_n_dot = R_nb * f_b + g_n;

R_nb_dot = R_nb * Skew;

== matlab function Copy_3_continuos_plant/Translational Motion Observer/Riccati_Equation/A1 ==
  data: A output
function A = A()

 A = zeros(10);

A(1:3,5:7) = eye(3);
A(5:7,8:10) = eye(3);
 

% A = eye(10);

end

== matlab function Copy_3_continuos_plant/Attitude Observer/b_computation ==
  data: J input; b_dot_stim output size=3; Kp input; ki input; t input; R_nb_stim input; b_stim input
function b_dot_stim  = b_dot_stim_func(J, Kp, ki, t, R_nb_stim, b_stim)


%b_dot_stim = zeros(3 ,1);

% if t <= 1
%     R_nb_stim = eye(3);
% %      b_stim = zeros(3, 1);
% %     
% end

SAT = sat(R_nb_stim)';
PA = pa( SAT * Kp * J);
VEX = vexfunc(PA);
b_dot_stim = Proj(b_stim , -ki * VEX);
% b_dot_stim = Proj(-ki * VEX, 0.5);

end

== matlab function Copy_3_continuos_plant/Translational Motion Observer/translation_motion_observer Function ==
  data: delta input; C_dx input; K input; beta_dot_stim output; J_stim input; R_nb_stim input; p_n_delta_dot_stim output; v_n_dot_stim output; f_n_stim output size=[3,1]; v_n_stim input size=3; f_b_imu input size=3; beta_stim input; p_n_delta_stim input size=3; sigma input; K_p input; epsilon_dot output; epsilon input size=3; t input
function [beta_dot_stim,p_n_delta_dot_stim,v_n_dot_stim,f_n_stim,epsilon_dot] =  TMO_func(delta,C_dx,K,J_stim,R_nb_stim, v_n_stim,f_b_imu, beta_stim, p_n_delta_stim,sigma,K_p,epsilon,t)

%obtained by Riccati equation
 K_pp = K(1:3,:); 
 K_beta_p = K(4,:);
 K_v_p = K(5:7,:);
 K_eps_p = K(8:10,:);

% remember to insert a clock to define dimensions of all variables
g_n = [0.1 0.1 9.81]';

if(t == 0) 
    delta_stim = zeros(3, 1);
    delta_diff = zeros(3, 1);
    v_n_stim = zeros(3, 1);
%     beta_stim = 0;
    epsilon = zeros(3,1);
    p_n_delta_stim = zeros(3, 1);
        
end



x_stim = [p_n_delta_stim; beta_stim];
%delta_stim = 2*C_dx*x_stim;
%delta_diff = (delta - delta_stim);



p_n_delta_dot_stim = v_n_stim + K_pp * (delta - 2*C_dx*x_stim);       % eq 14


beta_dot_stim = K_beta_p * (delta - 2*C_dx*x_stim);                       % eq 15

f_n_stim = R_nb_stim * f_b_imu + epsilon ;         % eq 18


v_n_dot_stim  = f_n_stim + g_n + K_v_p*(delta - 2*C_dx*x_stim);         % eq 16


epsilon_dot   = -sigma * K_p * J_stim * f_b_imu + K_eps_p * (delta - 2*C_dx * x_stim); % eq 17

end

== matlab function Copy_3_continuos_plant/Nonlinear algebraic transform and solution/Computation of Cdx ==
  data: y input; p_n_i input; C_dx output size=[6,4]
function C_dx  = C_dx_func(y,p_n_i)

    % y vector 
    % p matrix has row vectors
    %            (x,y,z) cols 
    %            m-rows are transponders number
    % all variables are in navigation frame oh yeah! baby ;)
    
    [row,col] = size(p_n_i);
    [row_,col_] = size(y);
    
    % m-measure vector
    p_m = p_n_i(row,:); % measure of m-th transponder
    y_m = y(row_);  % m-th pseudorange measure

    m = row; % m is transpoders number
    
    
    p_ = zeros(m-1,3); %row vector, 3 stands for x,y,z
    y_ = zeros(m-1,1);
    
    for i = 1 : 1 : m-1
    
        p_(i,:) = p_m - p_n_i(i,:);
        y_(i) = y(i) - y_m;
        
    end
    
    C_dx = [p_, y_];

end

== matlab function Copy_3_continuos_plant/Nonlinear algebraic transform and solution/Computation of delta ==
  data: y input; delta output size=6; p input; p0 input
function delta   = delta_func(y, p, p0)

    % y vector 
    % p matrix has row vectors
    %            (x,y,z) cols 
    %            m-rows are the numbers of the transponders
    % all variables are in navigation frame oh yeah! baby ;)
    % z is a col vector of scalars
    
    % we must choose p0 (a block)
    
    [row,col] = size(p);
    %[row_,col_] = size(y);
    
    p_los = zeros(row,col);
    z = zeros(row,1);   % dim = m x 1
    
    %defining los vector
    for i = 1:1:row
       p_los(i,:) = p(i,:) - p0';       % dim = m x 3
    end
    
%     p_n_true = p_los;
    
    % p_los = p_los';
    
    for i = 1:1:row
        z(i)= ((y(i)^2) - norm(p_los(i,:))^2); % dim = m x 1
    end
    
%     z = z';
%     
%     delta = zeros(row-1,1);
%     z_m = z(end);
%     
%     for i = 1:1:row-1
%         delta(i) =  (z(i) - z_m); %amm fenito
%     end

    delta = zeros(row-1,1); %dim = (m-1) x 1
    z_m = z(row,1);
    
    for i=1:1:(row-1)
        delta(i,1) = z(i,1) - z_m;
    end

end

== matlab function Copy_3_continuos_plant/Translational Motion Observer/Riccati_Equation/MATLAB Function2 ==
  data: A input; y output; P input
function y = fcn(A,P)

y = P * A;

end

== matlab function Copy_3_continuos_plant/Translational Motion Observer/Riccati_Equation/MATLAB Function3 ==
  data: A input; y output; P input
function y = fcn(A,P)

y = A' * P;

end

== matlab function Copy_3_continuos_plant/Translational Motion Observer/Riccati_Equation/MATLAB Function4 ==
  data: P input; y output; Ctrasp input; Rinv input
function y = fcn(P, Ctrasp, Rinv)

y = P * Ctrasp * Rinv;

end

== matlab function Copy_3_continuos_plant/Attitude Observer/Rot_func ==
  data: b_stim input; R_nb_stim_dot output; w_ib input; sigma input; Kp input; J input; R_nb_stim input; Skew output
function [R_nb_stim_dot, Skew] = rot_func(b_stim,w_ib,sigma,Kp,J,R_nb_stim) 

Skew = skew(w_ib - b_stim);

R_nb_stim_dot = R_nb_stim * Skew + sigma * Kp * J;

== matlab function Copy_3_continuos_plant/Kalman - Bucy Filter/Correction ==
  data: x_k_ input; H input; R input size=[6,6]; P_k_ input size=[10,10]; z_k input; x_k output; P_k output
function [x_k, P_k]  = correction(x_k_ , H, R, P_k_ ,z_k)

    n = size(P_k_);
    
%     P_k = zeros(10,10);


    K_k = P_k_ * H' * pinv(H * P_k_ * H' + R);
    
    x_k = x_k_ + K_k * (z_k - H * x_k_);
    
    P_k = (eye(n) - K_k * H) * P_k_;

end

== matlab function Copy_3_continuos_plant/Attitude Observer/MATLAB Function2 ==
  data: u input; y output
function y = fcn(u)

y = norm(u);

== matlab function Copy_3_continuos_plant/Translational Motion Observer/Riccati_Equation/C_ ==
  data: C output; C_dx input size=[6,4]
function C = C(C_dx)

   row = size(C_dx,1); 

 C1 = zeros(row,6);
 C = [2*C_dx C1];
 

% C1 = zeros(row, 2);
% 
% C = [C_dx C_dx C1];

== matlab function Copy_3_continuos_plant/Translational Motion Observer/A ==
  data: A output
function A = A()

 A = zeros(10);

 A(1:3,5:7) = eye(3);
 A(5:7,8:10) = eye(3);
 
end

== matlab function Copy_3_continuos_plant/Translational Motion Observer/C ==
  data: C output; C_dx input
function C = Cfunc(C_dx)

   row = size(C_dx,1); 

   C1 = zeros(row,6);

 C = [2*C_dx C1];
 
 
end

== matlab function Copy_3_continuos_plant/Translational Motion Observer/B_ ==
  data: B_ output
function B_ = B()

 B_ = zeros(10,3);

 B_(8:10,1:3) = eye(3);
end

== matlab function Copy_3_continuos_plant/Translational Motion Observer/Riccati_Equation/P_matrix  ==
  data: P output
function P = P()

P = eye(10);
 
%  P = diag([3 * 10^3,3 * 10^3,3 * 10^3,3 * 10^3,10,10,10,0.01,0.01,0.01]);
 
end

== matlab function Copy_3_continuos_plant/pseudorange_measurement_model ==
  data: p_n input; y output size=[7,1]; p_n_i input; beta input; epsilon input
function y = pseudorange_mea_model(p_n, p_n_i, beta, epsilon)

  %  row-vector

  y = zeros(size(p_n_i,1),1);

  for i = 1:1:size(p_n_i,1)

      rho = norm(p_n - (p_n_i(i,:))');  % eq. 7
      
      y(i) = rho + beta + epsilon(i); % eq. 8 

  end
      
end

== matlab function Copy_3_continuos_plant/Translational Motion Observer/Riccati_Equation/switch_function ==
  data: P1 input; P output; clock input; P2 input
function P = switch_function(P1, clock, P2)

if clock == 0
    P = P1;
else
    P = P2;
end

end

== matlab function Copy_3_continuos_plant/Translational Motion Observer/Riccati_Equation/MATLAB Function5 ==
  data: u input; y output
function y = fcn(u)


y = norm(u);

== matlab function Copy_3_continuos_plant/Local linearization1/linearisation ==
  data: K input size=[10,6]; AL output size=[10,10]; BL output size=[10,3]; CL output size=[6,10]; C input size=[6,10]; A input size=[10,10]; B input size=[10,3]; p_n_delta_stim input size=[3,1]; v_n_stim input size=[3,1]; f_n_stim input size=[3,1]; f_b_imu input size=[1,3]; beta_stim input size=1
function [AL, BL, CL] = linearisation(K,C,A,B, p_n_delta_stim, v_n_stim, f_n_stim, f_b_imu, beta_stim)

 % building state vector
 % xsi = [p_n_stim ; beta_stim; v_n_stim; f_n_tim];
%   xsi = zeros(10,1);
%   xsi(1:3,1) = p_n_delta_stim;
%   xsi(4,1) = beta_stim;
%   xsi(5:7,1) = v_n_stim;
%   xsi(8:10,1) = f_n_stim;
 % coder.extrinsic('ss');
 % sys = ss(A-K*C,B,C,0);
% % getting work point
%coder.extrinsic('trim');
%[X,U,Y,DX] = trim('sys', xsi);

% computing linearisation model
%coder.extrinsic('linmod');
%[AL, BL, CL, DL] = linmod('sys',X,U);

  
AL = zeros(10,10);
BL = zeros(10,3);
CL = zeros(size(C,1), 10);


coder.extrinsic('LinearizationFun');

[Al,Bl,Cl] = LinearizationFun(K,C,A,B);

p_n0 = p_n_delta_stim(1,1);
p_n1 = p_n_delta_stim (2,1);
p_n2 = p_n_delta_stim(3,1);

v_n0 = v_n_stim(1,1);
v_n1 = v_n_stim(2,1);
v_n2 = v_n_stim(3,1);

f_n0 = f_n_stim(1,1);
f_n1 = f_n_stim(2,1);
f_n2 = f_n_stim(3,1);

f_b0 = f_b_imu(1,1);
f_b1 = f_b_imu(1,2);
f_b2 = f_b_imu(1,3);


coder.extrinsic('eval');

AL_ = eval(Al);
BL_ = eval(Bl);
CL_ = eval(Cl);

% AL_ = feval('Al', p_n0, p_n1, p_n2,v_n0, v_n1, v_n2, f_n0, f_n1, f_n2, beta_stim);
% BL_ = feval('Bl', f_b0, f_b1, f_b2);
% CL_ = feval('Cl', p_n0, p_n1, p_n2,v_n0, v_n1, v_n2, f_n0, f_n1, f_n2, beta_stim);
% 

AL = AL_;
BL = BL_;
CL = CL_;


end

== matlab function Copy_3_continuos_plant/Attitude Observer/from body to NED frame ==
  data: m_b_mag input; t input; R_bn input; m_n_mag output
function m_n_mag = b2n(m_b_mag, t, R_bn)

% m_n_mag and m_b_mag are 3x1

if t==0
    R_bn = eye(3);
end

m_n_mag = R_bn * m_b_mag;

== matlab function Copy_3_continuos_plant/Attitude Observer/matrixInverse ==
  data: A input; AInv output
function AInv  = matrixInverse(A)

% inverse by singular value decomposition


[n,m] = size(A);

% U = zeros(n,n);
% V = zeros(n,n);
% S = zeros(n,n);

[U,S,V] = svd(A);

pos = 0;

% maximun admissible condition number
csi = 10^3;

for i=n:-1:1
    if( S(1,1)/S(i,i) > csi)
        S(i,i) = 0;
        pos = i; % keeps the last eliminated singular value
    end
end

tempS = S(1:pos-1,1:pos-1); %take the non-zero set
tempS = inv(tempS);
S(1:pos-1,1:pos-1) = tempS(1:pos-1,1:pos-1); % now S is the inverse matrix
AInv = V * S * U';

end

== matlab function Copy_3_continuos_plant/Translational Motion Observer/Riccati_Equation/MATLAB Function6 ==
  data: u input; y output
function y = fcn(u)

y = norm(u);

== matlab function Copy_3_continuos_plant/Translational Motion Observer/Riccati_Equation/MATLAB Function7 ==
  data: clock input; y output; A input; C input; K input
function y = fcn(clock, A, C, K)

% if clock <= 20
    y = A;
% else
%     y = A - K*C;
% % end
end

== matlab function Copy_3_continuos_plant/Translational Motion Observer/Riccati_Equation/MATLAB Function8 ==
  data: y output
function y = myPlacement()

C =  1000*   [ -1.5000    1.2000         0    0.3000         0         0         0         0  0 0;
         0   -0.8000   -0.0100    0.8001         0         0         0         0    0 0;
   -3.0000   -0.8000   -0.0400    2.4059         0         0         0         0    0 0;
   -3.0000    1.2000   -0.0200    1.8001         0         0         0         0    0 0;
   -1.5000   -0.8000   -0.0300    1.3003         0         0         0         0    0 0];



K = [    10     0     0     0     0;
     0    10     0     0     0;
     0     0    10     0     0;
     0     0     0    10     0;
     0     0     0     0    10;
    10     0     0     0     0;
     0    10     0     0     0;
     0     0    10     0     0;
     0     0     0    10     0;
     0     0     0     0    10];
 
 
 y = K * C;
   
   

end

== matlab function Copy_3_continuos_plant/Translational Motion Observer/Riccati_Equation/MATLAB Function9 ==
  data: y output; A input; CK input; t input
function y = oneFun(A, CK, t)

% if t <= 1
    y = A - CK;
% else
%     y = A;

   

end

== matlab function Copy_3_continuos_plant/Translational Motion Observer/Riccati_Equation/MATLAB Function10 ==
  data: y output
function y = myGain()

Gain = 1000 * [-1.0308    0.2080   -2.1181   -1.7236   -1.1219;
    1.5540   -0.9782   -1.4402    1.6629   -1.3249;
    1.0278   -2.1284    0.2466   -2.0553   -0.4035;
   -0.1547    0.3620   -0.0435    0.2578   -0.0733;
   -0.0200   -0.3758   -0.8435    0.1880    0.3340;
   -0.6041    0.2009   -0.0138   -0.5953    0.4901;
    0.1845   -0.2811    0.4856    0.3175    0.7418;
   -0.0018    0.0037   -0.0011    0.0037    0.0006;
    0.0004   -0.0011    0.0003   -0.0012    0.0001;
    0.0026   -0.0054    0.0013   -0.0052   -0.0005]

y = Gain;

== matlab function Copy_3_continuos_plant/Translational Motion Observer/Riccati_Equation/myC ==
  data: C output
function C = myC()
% 
% C = 1000 * [  -1.5000    1.2000         0    0.3000         0         0         0         0         0   0;
%          0   -0.8000   -0.0100    0.8001         0         0         0         0         0  0;
%    -3.0000   -0.8000   -0.0400    2.4059         0         0         0         0         0  0;
%    -3.0000    1.2000   -0.0200    1.8001         0         0         0         0         0  0;
%    -1.5000   -0.8000   -0.0300    1.3003         0         0         0         0         0  0];
% 
%  
C = zeros(6,10);
C(1:6,1:6) = eye(6);
C(1:3,7:9) = eye(3);
C(4:6,7:9) = eye(3);
end

== matlab function Copy_3_continuos_plant/Mechanisation subsystem/from angular velocity to euler angles ==
  data: w_ib input; phi input; theta input; psi input; phi_dot output; theta_dot output; psi_dot output
function [phi_dot, theta_dot, psi_dot] = w2doteuler(w_ib, phi, theta, psi)


D = zeros(3,3);
D(1,1) = 1;
D(1,2) = sin(phi)*tan(theta);
D(1,3) = cos(phi)*tan(theta);

D(2,2) = cos(phi);
D(2,3) = -sin(phi);

D(3,2) = sin(phi)/cos(theta);
D(3,3) = cos(phi)/cos(theta); 


% D = [ 1    sin(phi)*tan(theta)     cos(phi)*tan(theta);
%       0        cos(phi)                - sin(phi);
%       0    sin(phi)/cos(theta)     cos(phi)/cos(theta)]; 

phi_dot = D(1,:) * w_ib;
theta_dot = D(2,:) * w_ib;
psi_dot = D(3,:) * w_ib;

end

== matlab function Copy_3_continuos_plant/Mechanisation subsystem/MATLAB Function ==
  data: phi input; R output; theta input; psi input
function R = eul2R(phi, theta, psi)

angles = [phi theta psi];

R = eul2rotm(angles,'ZYX');

end

== matlab function Copy_3_continuos_plant/Mechanisation subsystem/MATLAB Function1 ==
  data: u input; y output
function y = fcn(u)

y = norm(u);

== matlab function Copy_3_continuos_plant/Mechanisation subsystem/mechanisation ==
  data: f_b_imu input; v_n_dot output; R_nb input
function v_n_dot  = mechanisation(f_b_imu, R_nb)

g_n = [0.1 0.1 9.81]';

v_n_dot = R_nb * f_b + g_n;

end

== matlab function Copy_3_continuos_plant/Attitude Observer/MATLAB Function ==
  data: u input; y output
function y = fcn(u)

y = norm(u);

== matlab function Copy_3_continuos_plant/Attitude Observer/MATLAB Function1 ==
  data: phi input; R output; theta input; psi input
function R = eul2R(phi, theta, psi)

angles = [phi theta psi];

R = eul2rotm(angles,'ZYX');

end

== matlab function Copy_3_continuos_plant/Attitude Observer/from angular velocity to euler angles ==
  data: w_ib input; phi input; theta input; psi input; phi_dot output; theta_dot output; psi_dot output
function [phi_dot, theta_dot, psi_dot] = w2doteuler(w_ib, phi, theta, psi)


D = zeros(3,3);
D(1,1) = 1;
D(1,2) = sin(phi)*tan(theta);
D(1,3) = cos(phi)*tan(theta);

D(2,2) = cos(phi);
D(2,3) = -sin(phi);

D(3,2) = sin(phi)/cos(theta);
D(3,3) = cos(phi)/cos(theta); 


% D = [ 1    sin(phi)*tan(theta)     cos(phi)*tan(theta);
%       0        cos(phi)                - sin(phi);
%       0    sin(phi)/cos(theta)     cos(phi)/cos(theta)]; 

phi_dot = D(1,:) * w_ib;
theta_dot = D(2,:) * w_ib;
psi_dot = D(3,:) * w_ib;

end

== matlab function Copy_3_continuos_plant/Translational Motion Observer/Riccati_Equation/MATLAB Function11 ==
  data: u input; y output
function y = fcn(u)

y = norm(u);

== matlab function Copy_3_continuos_plant/Translational Motion Observer/Riccati_Equation/MATLAB Function12 ==
  data: u input; y output
function y = fcn(u)

y = norm(u(1:8,1:8));

== matlab function Copy_3_continuos_plant/Translational Motion Observer/Riccati_Equation/MATLAB Function13 ==
  data: u input; y output
function y = fcn(u)

y = norm(u);

== matlab function Copy_3_continuos_plant/Translational Motion Observer/Riccati_Equation/MATLAB Function14 ==
  data: u input; y output
function y = fcn(u)

y = norm(u);

== matlab function Copy_3_continuos_plant/Attitude Observer/MATLAB Function3 ==
  data: u input; y output
function y = fcn(u)

y = norm(u);

== matlab function Copy_3_continuos_plant/Translational Motion Observer/Riccati_Equation/MATLAB Function16 ==
  data: u input; y output
function y = fcn(u)

y = norm(u);
